simulink model "linearisation"  (R2023b)
settings: Solver=VariableStepAuto  StartTime=0.0  StopTime=100  MaxStep=1e-4  RelTol=1e-3
settings Model: Creator=33783  LastModifiedBy=33783

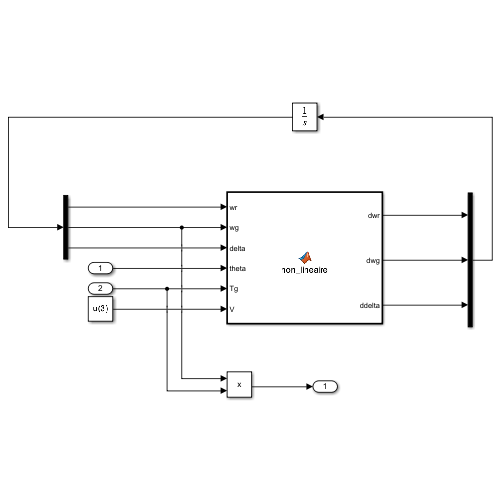
[thumbnail: Simulink's stored preview of the top-level diagram]
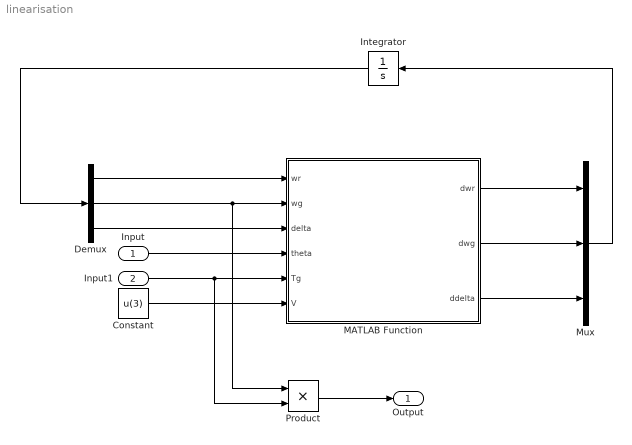
== system linearisation ==
  Input : Inport
  Input1 : Inport  Port=2
  Constant : Constant  Value=u(3)
  Demux : Demux  Outputs=3
  Integrator : Integrator
  MATLAB Function : MATLAB Function  TreatAsAtomicUnit=on
  Mux : Mux  Inputs=3
  Product : Product
  Output : Outport
  wires:
  Mux/1 -> Integrator/1
  MATLAB Function/1(dwr) -> Mux/1
  MATLAB Function/2(dwg) -> Mux/2
  Demux/1 -> MATLAB Function/1(wr)
  Demux/2 -> Product/1, MATLAB Function/2(wg)
  Demux/3 -> MATLAB Function/3(delta)
  MATLAB Function/3(ddelta) -> Mux/3
  Integrator/1 -> Demux/1
  Input/1 -> MATLAB Function/4(theta)
  Input1/1 -> Product/2, MATLAB Function/5(Tg)
  Constant/1 -> MATLAB Function/6(V)
  Product/1 -> Output/1

== matlab function linearisation/MATLAB Function ==
  data: wr input; dwr output; wg input; delta input; theta input; Tg input; dwg output; ddelta output; V input
function [dwr,dwg,ddelta] = non_lineaire(wr,wg,delta,theta,Tg,V)
    %% Représentation d'état non linéaire :
    % Valeurs du modèle :
    n_g = 43.165 ; % sans unité
    J_r = 3.25e5 ; % kg/m^2
    J_g = 34.4 ; % kg/m^2
    K_s = 269.1e3 ; % N.m/rad
    R = 21.65 ; % en mètres
    rho = 1.292 ; % en kg/m3
  
    D_s= 9500; % Nm/rad/s
    
   
    function Lambdai = funLambdai(lambda,theta)
        Lambdai = 1/(1/(lambda+0.08*theta)- 0.035/(theta^3 + 1)) ;
    end
    
    function Cp = funCp(lambda,theta) 
        Cp = 0.5*(116/funLambdai(lambda,theta)-0.4*theta-5)*exp(-21/funLambdai(lambda,theta)) + 0.0068*lambda ;
    end
    
    % Puissance 
    function Pr = funPuissance(wr,theta,V)
        lambda=(wr*R)/V;
        Pr = 0.5*rho*pi*(R^2)*(V^3)*funCp(lambda,theta);
    end
    
    dwr = 1/(J_r*wr) * funPuissance(wr,theta,V) - (D_s/J_r) * wr + (D_s/(J_r*n_g)) * wg - (K_s/J_r) * delta ;
    dwg = (D_s/(J_g * n_g)) * wr - (D_s/(J_g * n_g^2)) * wg + (K_s/(J_g * n_g)) * delta - (1/J_g) * Tg ;
    ddelta = wr - 1/n_g * wg;

    end
